simulink model "sampleModel1580_3_sub"  (R2023a)
settings: Solver=VariableStepAuto  StartTime=0.0  StopTime=10.0  RelTol=1e-3
libraries: hdlsllib x6, simulink x2
settings Model: Creator=user1  LastModifiedBy=user1
settings OptimizationCC: BlockReduction=off  ConditionallyExecuteInputs=off

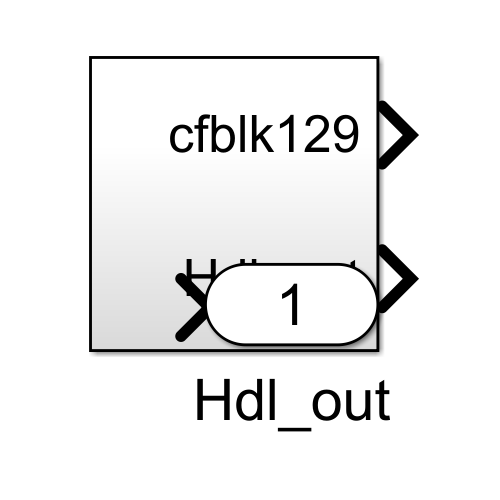
[thumbnail: Simulink's stored preview of the top-level diagram]
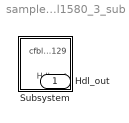
== system sampleModel1580_3_sub ==
  Subsystem : Subsystem
  Hdl_out : Outport  OutDataTypeStr=uint8

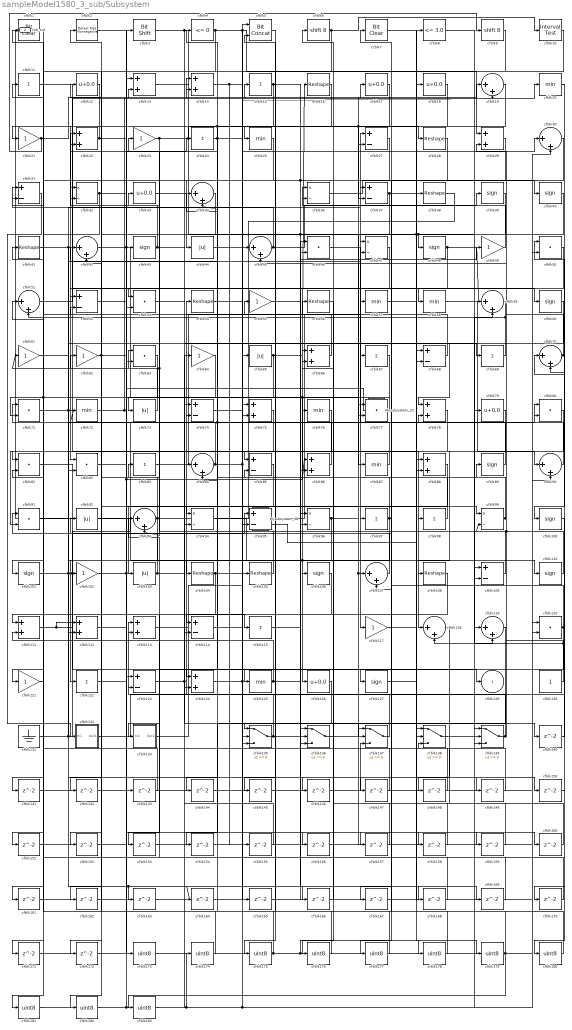
== system sampleModel1580_3_sub/Subsystem ==
  Mysubsystem_23 : Subsystem  TreatAsAtomicUnit=on  RTWFcnName=Mysubsystem_23
      settings: RTWFcnNameOpts=User specified  RTWFileNameOpts=Use function name
  Mysubsystem_38 : Subsystem  TreatAsAtomicUnit=on  RTWFcnName=Mysubsystem_38
      settings: RTWFcnNameOpts=User specified  RTWFileNameOpts=Use function name
  cfblk1 : simulink/Logic and Bit Operations/Bit Clear  iBit=0
      settings: LibrarySourceBlock=|
      | hdlsllib/Logic and Bit
      | Operations/Bit Clear
  cfblk10 : hdlsllib/Logic and Bit Operations/Interval Test  IntervalClosedRight=on  uplimit=0.5  IntervalClosedLeft=on  lowlimit=-0.5  OutDataTypeStr=uint8
  cfblk{39..40,43,48,60,89,100..101,106,110,127} (11 alike) : Signum
  cfblk{21,23,49,55,61..62,64,102,117,121} (10 alike) : Gain  OutDataTypeStr=uint8
  cfblk{44,65,73,92,103} (5 alike) : Abs  OutDataTypeStr=uint8  SaturateOnIntegerOverflow=off
  cfblk{16,28,38,41,54,56,104..105,108} (9 alike) : Reshape
  cfblk{19,30,34,42,45,51,59,70,84,90,93,107,118..119} (14 alike) : Sum  Inputs=|++  OutDataTypeStr=uint8
  cfblk{27,31,37,52,68,74,85,95,109,114,123} (11 alike) : Sum  Inputs=+-  OutDataTypeStr=uint8
  cfblk{11,15,24,67,69,83,97..98,115,122} (10 alike) : Sum  Inputs=+  OutDataTypeStr=uint8
  cfblk{13..14,22,29,66,75,78,86,88,111..113,124} (13 alike) : Sum  OutDataTypeStr=uint8
  cfblk{12,17..18,33,79,126} (6 alike) : Bias  Bias=0.0  SaturateOnIntegerOverflow=off
  cfblk{46,50,53,63,71,77,80..82,91,120} (11 alike) : DotProduct  OutDataTypeStr=uint8
  cfblk{20,25,57..58,72,76,87,125} (8 alike) : MinMax  OutDataTypeStr=uint8
  cfblk130 : Constant  OutDataTypeStr=uint8  SampleTime=-1
  cfblk131 : Ground
  cfblk132 : Subsystem
      settings: LibrarySourceBlock=|
      | hdlsllib/Ports &
      | Subsystems/Subsystem
  cfblk133 : Subsystem
      settings: LibrarySourceBlock=|
      | hdlsllib/Ports &
      | Subsystems/Subsystem
  cfblk{135..139} (5 alike) : Switch  OutDataTypeStr=uint8  SaturateOnIntegerOverflow=off  InputSameDT=off
  cfblk{140..172} (33 alike) : Delay  SampleTime=1
  cfblk{173..183} (11 alike) : DataTypeConversion  OutDataTypeStr=uint8  SaturateOnIntegerOverflow=off  RndMeth=Floor
  cfblk2 : hdlsllib/Logic and Bit Operations/Detect Rise Nonnegative  vinit=0  OutDataTypeStr=uint8
  cfblk3 : hdlsllib/Logic and Bit Operations/Bit Shift  mode=Shift Left Logical  N=0
  cfblk{32,36,47,94,96,99} (6 alike) : Product  Inputs=*/  OutDataTypeStr=uint8  RndMeth=Zero  SaturateOnIntegerOverflow=on
  cfblk4 : hdlsllib/Logic and Bit Operations/Compare To Zero  relop=<=  OutDataTypeStr=uint8
  cfblk5 : hdlsllib/Logic and Bit Operations/Bit Concat  numInputs=2
  cfblk6 : ArithShift  BitShiftNumber=8
  cfblk7 : simulink/Logic and Bit Operations/Bit Clear  iBit=0
      settings: LibrarySourceBlock=|
      | hdlsllib/Logic and Bit
      | Operations/Bit Clear
  cfblk8 : hdlsllib/Logic and Bit Operations/Compare To Constant  relop=<=  const=3.0  OutDataTypeStr=uint8
  cfblk9 : ArithShift  BitShiftNumber=8
  cfblk129 : Outport  OutDataTypeStr=uint8  VectorParamsAs1DForOutWhenUnconnected=off
  Hdl_out : Outport  Port=2  OutDataTypeStr=uint8
  wires:
  cfblk83/1 -> cfblk55/1
  cfblk77/1 -> cfblk73/1
  cfblk81/1 -> cfblk125/1
  cfblk72/1 -> cfblk158/1, cfblk15/1
  cfblk94/1 -> cfblk110/1
  cfblk132/1(Out1) -> cfblk50/1
  cfblk135/1 -> cfblk147/1, cfblk54/1
  cfblk137/1 -> cfblk113/1
  cfblk4/1 -> cfblk114/2, cfblk19/2, cfblk29/1
  cfblk103/1 -> cfblk140/1, cfblk32/1
  cfblk58/1 -> cfblk90/1
  cfblk24/1 -> cfblk96/2, cfblk104/1
  cfblk29/1 -> cfblk145/1, cfblk46/2
  cfblk36/1 -> cfblk40/1
  cfblk32/1 -> cfblk141/1, cfblk77/2
  cfblk11/1 -> cfblk58/1
  cfblk22/1 -> cfblk169/1, cfblk21/1
  cfblk71/1 -> cfblk85/1, cfblk164/1, cfblk163/1
  cfblk5/1 -> cfblk175/1
  cfblk6/1 -> cfblk172/1, cfblk10/1
  cfblk39/1 -> cfblk177/1, cfblk68/2
  cfblk107/1 -> cfblk92/1
  cfblk23/1 -> cfblk93/2, cfblk119/2, cfblk28/1
  cfblk19/1 -> cfblk94/1
  cfblk45/1 -> cfblk31/1, cfblk39/1
  cfblk14/1 -> cfblk156/1, cfblk155/1
  cfblk133/1(Out1) -> cfblk65/1
  cfblk12/1 -> cfblk82/1
  cfblk42/1 -> cfblk14/1, cfblk126/1
  cfblk46/1 -> cfblk117/1
  cfblk86/1 -> cfblk63/1
  cfblk9/1 -> cfblk81/1
  cfblk65/1 -> cfblk102/1, cfblk16/1
  cfblk127/1 -> cfblk8/1
  cfblk111/1 -> cfblk112/1, cfblk95/1
  cfblk21/1 -> cfblk13/2, cfblk9/1
  cfblk57/1 -> cfblk60/1
  cfblk104/1 -> cfblk152/1, cfblk75/1
  cfblk16/1 -> cfblk25/1
  cfblk41/1 -> cfblk149/1, cfblk118/1
  cfblk49/1 -> cfblk36/1
  cfblk78/1 -> cfblk98/1
  cfblk25/1 -> cfblk44/1
  cfblk117/1 -> cfblk18/1
  cfblk122/1 -> cfblk3/1
  cfblk90/1 -> cfblk27/1
  cfblk7/1 -> cfblk179/1
  cfblk20/1 -> cfblk70/2
  cfblk68/1 -> cfblk11/1
  cfblk34/1 -> cfblk94/2
  cfblk67/1 -> cfblk76/1, cfblk124/1
  cfblk30/1 -> cfblk127/1
  cfblk59/1 -> cfblk82/2, cfblk51/2
  cfblk105/1 -> cfblk61/1, cfblk33/1
  cfblk91/1 -> cfblk47/1
  cfblk124/1 -> cfblk159/1, cfblk56/1
  cfblk3/1 -> cfblk69/1, cfblk105/1
  cfblk131/1 -> cfblk80/2, cfblk38/1
  cfblk50/1 -> cfblk97/1
  cfblk95/1 -> cfblk47/2
  cfblk28/1 -> cfblk111/1
  cfblk93/1 -> cfblk52/2, cfblk122/1
  cfblk79/1 -> cfblk95/2
  cfblk109/1 -> cfblk4/1
  cfblk89/1 -> cfblk6/1
  cfblk113/1 -> cfblk115/1
  cfblk66/1 -> cfblk23/1
  cfblk125/1 -> cfblk168/1, cfblk111/2
  cfblk51/1 -> cfblk20/1
  cfblk73/1 -> cfblk62/1
  cfblk27/1 -> cfblk53/1
  cfblk44/1 -> cfblk30/1
  cfblk13/1 -> cfblk75/2
  cfblk97/1 -> cfblk167/1, cfblk114/1, cfblk22/2
  cfblk138/1 -> cfblk109/2
  cfblk52/1 -> cfblk13/1
  cfblk136/1 -> cfblk19/1, cfblk107/1
  cfblk120/1 -> cfblk91/1, cfblk133/1(In1), cfblk118/2
  cfblk15/1 -> cfblk157/1, cfblk52/1
  cfblk101/1 -> cfblk166/1, cfblk136/2, cfblk86/1, Mysubsystem_23/1(In1)
  cfblk69/1 -> cfblk67/1
  cfblk55/1 -> cfblk57/1
  cfblk40/1 -> cfblk63/2, cfblk48/1
  cfblk74/1 -> cfblk17/1
  cfblk48/1 -> cfblk135/2, cfblk59/1
  cfblk53/1 -> cfblk88/2
  cfblk130/1 -> cfblk85/2
  cfblk123/1 -> cfblk136/3, cfblk84/1
  cfblk10/1 -> cfblk135/1
  cfblk18/1 -> cfblk37/2, cfblk124/2
  cfblk80/1 -> cfblk108/1
  cfblk115/1 -> cfblk49/1
  cfblk76/1 -> cfblk91/2
  cfblk99/1 -> cfblk29/2, cfblk66/1
  cfblk37/1 -> cfblk160/1, cfblk42/2, cfblk86/2
  cfblk70/1 -> cfblk100/1, cfblk45/2
  cfblk43/1 -> cfblk129/1, cfblk22/1
  cfblk17/1 -> cfblk34/2, cfblk101/1
  cfblk88/1 -> cfblk103/1
  cfblk96/1 -> cfblk78/2, cfblk112/2, cfblk106/1
  cfblk98/1 -> cfblk72/1, cfblk42/1
  cfblk60/1 -> cfblk78/1
  cfblk1/1 -> cfblk181/1
  cfblk84/1 -> cfblk71/1, cfblk80/1, cfblk137/2
  cfblk61/1 -> cfblk37/1
  cfblk33/1 -> cfblk87/1
  cfblk87/1 -> cfblk74/2
  cfblk31/1 -> cfblk132/1(In1)
  cfblk110/1 -> cfblk83/1
  cfblk92/1 -> cfblk138/1
  cfblk82/1 -> cfblk99/1
  cfblk102/1 -> cfblk150/1, cfblk24/1
  cfblk63/1 -> cfblk71/2, cfblk121/1
  cfblk139/1 -> cfblk123/2, cfblk99/2, cfblk89/1
  cfblk64/1 -> cfblk182/1
  cfblk62/1 -> cfblk14/2, cfblk12/1
  cfblk8/1 -> cfblk119/1
  cfblk140/1 -> cfblk70/1
  cfblk141/1 -> cfblk45/1
  cfblk47/1 -> cfblk142/1
  cfblk142/1 -> cfblk90/2
  cfblk112/1 -> cfblk143/1
  cfblk143/1 -> cfblk51/1
  cfblk119/1 -> cfblk144/1
  cfblk144/1 -> cfblk137/3
  cfblk145/1 -> cfblk109/1
  cfblk54/1 -> cfblk146/1
  cfblk146/1 -> cfblk27/2
  cfblk147/1 -> cfblk93/1
  cfblk118/1 -> cfblk148/1
  cfblk148/1 -> cfblk107/2
  cfblk149/1 -> cfblk46/1
  cfblk75/1 -> cfblk151/1
  cfblk151/1 -> cfblk53/2
  cfblk152/1 -> cfblk32/2
  cfblk106/1 -> cfblk153/1
  cfblk153/1 -> cfblk77/1
  cfblk126/1 -> cfblk154/1
  cfblk154/1 -> cfblk96/1
  cfblk155/1 -> cfblk74/1
  cfblk156/1 -> cfblk120/1
  cfblk157/1 -> cfblk137/1
  cfblk158/1 -> cfblk138/2
  cfblk159/1 -> cfblk138/3
  cfblk160/1 -> cfblk36/2
  cfblk121/1 -> cfblk161/1
  cfblk161/1 -> cfblk123/1
  cfblk85/1 -> cfblk162/1
  cfblk162/1 -> cfblk68/1
  cfblk163/1 -> cfblk59/2
  cfblk164/1 -> cfblk84/2
  cfblk114/1 -> cfblk165/1
  cfblk165/1 -> cfblk136/1
  cfblk166/1 -> cfblk66/2
  cfblk167/1 -> cfblk50/2
  cfblk168/1 -> cfblk81/2
  cfblk169/1 -> cfblk31/2
  cfblk100/1 -> cfblk170/1
  cfblk170/1 -> cfblk113/2
  cfblk108/1 -> cfblk171/1
  cfblk171/1 -> cfblk139/2
  cfblk172/1 -> cfblk139/1
  cfblk2/1 -> cfblk173/1
  cfblk173/1 -> cfblk79/1
  cfblk174/1 -> cfblk2/1
  cfblk175/1 -> cfblk34/1, cfblk178/1, cfblk120/2
  cfblk56/1 -> cfblk176/1
  cfblk176/1 -> cfblk5/1
  cfblk177/1 -> cfblk5/2
  cfblk178/1 -> cfblk7/1
  cfblk179/1 -> cfblk183/1, cfblk41/1
  cfblk150/1 -> cfblk180/1
  cfblk180/1 -> cfblk1/1
  cfblk181/1 -> cfblk139/3, cfblk43/1
  cfblk182/1 -> cfblk174/1, cfblk135/3, cfblk30/2
  cfblk183/1 -> cfblk64/1
  cfblk38/1 -> Mysubsystem_38/1(In1)
  Mysubsystem_38/1(Out1) -> Hdl_out/1, cfblk88/1

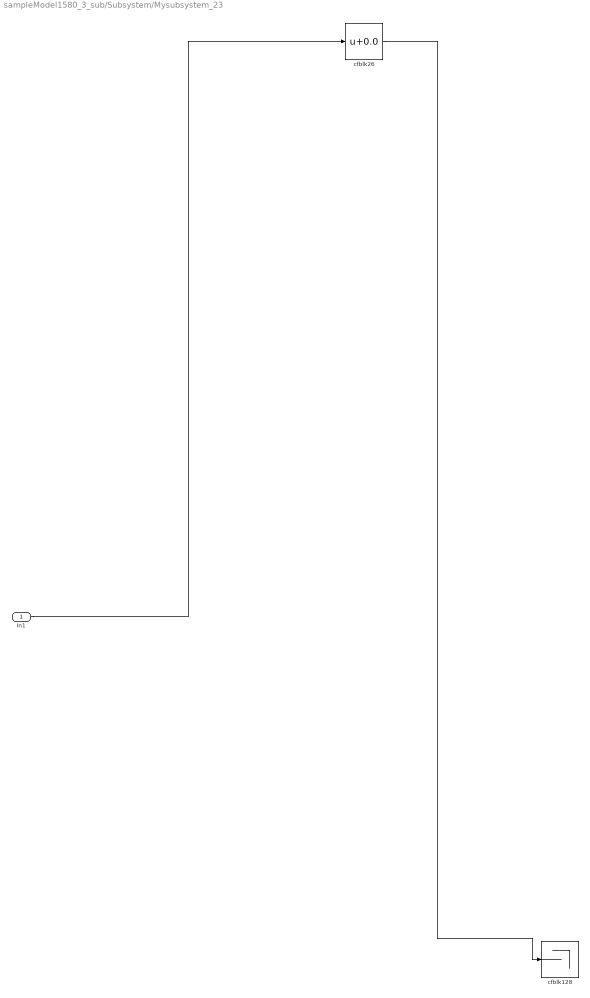
== system sampleModel1580_3_sub/Subsystem/Mysubsystem_23 ==
  In1 : Inport
  cfblk128 : Terminator
  cfblk26 : Bias  Bias=0.0  SaturateOnIntegerOverflow=off
  wires:
  In1/1 -> cfblk26/1
  cfblk26/1 -> cfblk128/1

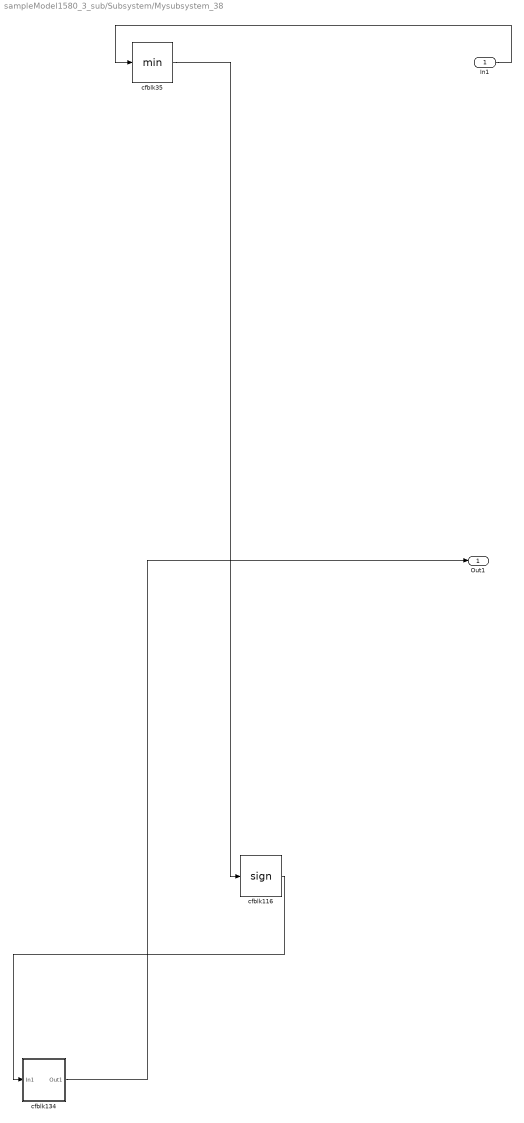
== system sampleModel1580_3_sub/Subsystem/Mysubsystem_38 ==
  In1 : Inport
  cfblk116 : Signum
  cfblk134 : Subsystem
      settings: LibrarySourceBlock=|
      | hdlsllib/Ports &
      | Subsystems/Subsystem
  cfblk35 : MinMax
  Out1 : Outport
  wires:
  In1/1 -> cfblk35/1
  cfblk35/1 -> cfblk116/1
  cfblk116/1 -> cfblk134/1(In1)
  cfblk134/1(Out1) -> Out1/1

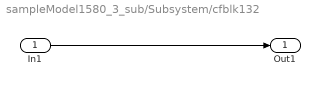
== system sampleModel1580_3_sub/Subsystem/cfblk132 ==
  In1 : Inport
  Out1 : Outport
  wires:
  In1/1 -> Out1/1

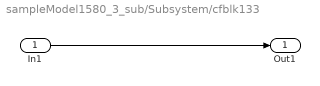
== system sampleModel1580_3_sub/Subsystem/cfblk133 ==
  In1 : Inport
  Out1 : Outport
  wires:
  In1/1 -> Out1/1

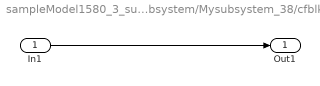
== system sampleModel1580_3_sub/Subsystem/Mysubsystem_38/cfblk134 ==
  In1 : Inport
  Out1 : Outport
  wires:
  In1/1 -> Out1/1
